simulink model "ev_control"  (R2024b)
settings: Solver=ode23t  StartTime=0  StopTime=3000  FixedStep=0.1  RelTol=1e-3
undefined symbols (not defined in the file or in its folder): DiscIntNeverNeededParam, Ion, Lithium
libraries: fl_lib x7, nesl_utility x7, sdl_lib x6, autolibshared x5, ee_lib x3, spsBatteryLib x1, spsControlledCurrentSourceLib x1, rllib x1, spspowerguiLib x1
settings Model: Creator=aaksh  LastModifiedBy=CSLAB

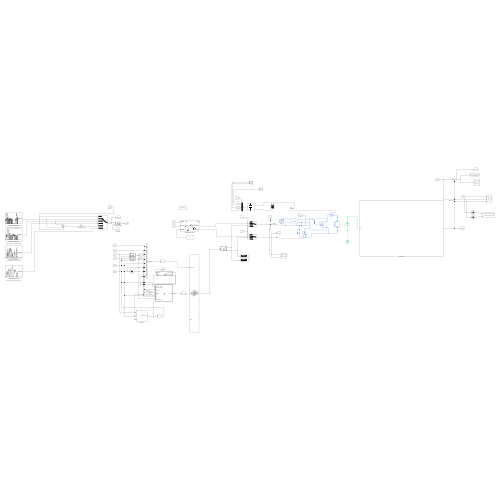
[thumbnail: Simulink's stored preview of the top-level diagram]
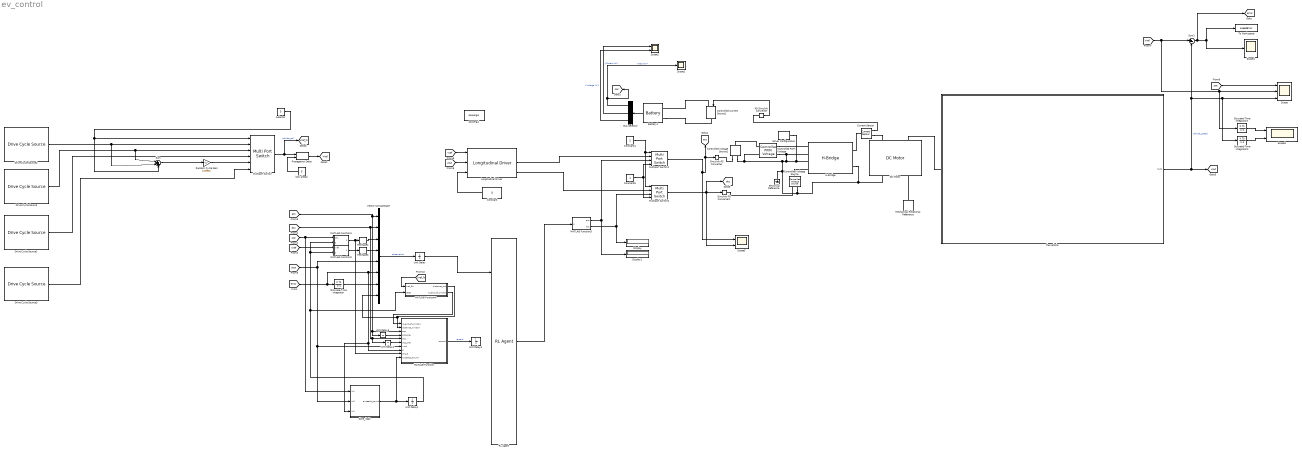
== system ev_control ==
  Battery1 : spsBatteryLib/Battery  BatType=Lithium-Ion  NomV=360  NomQ=77  SOC=76.3292  Batt_Tr=30  PresetModel=on  MaxQ=77  MinV=270  FullV=419.0354  Dis_rate=33.4783  R=0.046753  Normal_OP=69.6348  expZone="[388.9389      3.783043]"
      settings: LibrarySourceBlock=electricdrivelib/Extra Sources/Battery
  Bus Selector : BusSelector  OutputSignals=SOC (%),Current (A),Voltage (V)
  Constant : Constant  Value=0
  Constant4 : Constant  Value=2
  Constant5 : Constant
  Controlled Current Source1 : spsControlledCurrentSourceLib/Controlled Current Source  Initialize=on  Source_Type=AC  Amplitude=0  Phase=0  Frequency=0  Measurements=None
  Controlled PWM Voltage : ee_lib/Integrated Circuits/Controlled PWM Voltage  F=7 kHz  TD=0 s  pulse_width_offset=0 s  pulse_min=0 s  pwm_or_av=ee.enum.pwm_or_av.averaged  event_type=ee.enum.ic.event.asynchronous  sample_time=1e-6 s  Vmin=0 V  Vmax=1 V  Vm=1 V  u_min=0  u_max=1
  Controlled Voltage Source : fl_lib/Electrical/Electrical Sources/Controlled Voltage Source
  Controlled Voltage Source1 : fl_lib/Electrical/Electrical Sources/Controlled Voltage Source
  Current Sensor : fl_lib/Electrical/Electrical Sensors/Current Sensor
  DC Motor : ee_lib/Electromechanical/Brushed Motors/DC Motor  field_option=ee.enum.field_option.pm  Rf=100 Ohm  Lf=1 H  Laf=0.15 H  If0=0 A  parameterization=ee.enum.dcparam_option.load_speed  Ra=3.9 Ohm  La=100e-6 H  emf_or_torque=ee.enum.emf_or_torque.kv  Kv=0.072e-3 V/rpm  Ki=6.876e-4 N*m/A  T_stall=0.24e-3 N*m  w_max=8000 rpm  w_rated=6000 rpm  P_rated=89 kW  V_rated=360 V  lam_param=ee.enum.lam_param.damping  i_noload=0 A  V_i_noload=1.5 V  J=0.03 kg*m^2  lam=0.02 N*m*s/rad  speed0=0 rpm  t_fault_armature=1 s  t_fault_field=1 s  fault_action=simscape.enum.assert.action.none  alpha=3.93e-3 1/K  Tmeas=25 degC  thermal_mass=100 J/K  initial_temperature=25 degC
  Discrete-Time Integrator : DiscreteIntegrator  SampleTime=-1  ICPrevOutput=DiscIntNeverNeededParam  ICPrevScaledInput=DiscIntNeverNeededParam
  Discrete-Time Integrator1 : DiscreteIntegrator  SampleTime=-1  ICPrevOutput=DiscIntNeverNeededParam  ICPrevScaledInput=DiscIntNeverNeededParam
  Discrete-Time Integrator2 : DiscreteIntegrator  SampleTime=-1  ICPrevOutput=DiscIntNeverNeededParam  ICPrevScaledInput=DiscIntNeverNeededParam
  Display : Display
  Display1 : Display
  Drive Cycle Source : autolibshared/Drive Cycle Source  cycleVar=FTP72  fileVar=cycleFTP75.mat  tfinal="1372  seconds, Cyclic"  cycleRepeat=on  outAccPort=off  outGearPort=off  gearList=No gear data  t_wot1=5  xdot_woto=0  xdot_wot1=30  t_wot2=20  xdot_wot2=0  t_wotend=30  srcUnit=m/s  outUnit=m/s  srcAccUnit=m/s/s  outAccUnit=m/s^2  dt=0.1  aMode=1  faultOption=off  velBnd=2  velBndUnit=mph  inUnit=m/s  timeBnd=1  failOption=off  stopSim=off  maxFaultCnt=10  maxFaultTime=2  maxTotFaultTime=15  traceOption=off  dtTrace=1  traceWindow=10  lastDCname=FTP72  lastOutUnit=mph  lastDT=0  lastTB=1  lastSB=2  forceCalcBound=off
  Drive Cycle Source1 : autolibshared/Drive Cycle Source  cycleVar=NYCC  fileVar=cycleFTP75.mat  tfinal="598  seconds, Cyclic"  cycleRepeat=on  outAccPort=off  outGearPort=off  gearList=No gear data  t_wot1=5  xdot_woto=0  xdot_wot1=30  t_wot2=20  xdot_wot2=0  t_wotend=30  srcUnit=m/s  outUnit=m/s  srcAccUnit=m/s/s  outAccUnit=m/s^2  dt=0.1  aMode=1  faultOption=off  velBnd=2  velBndUnit=mph  inUnit=m/s  timeBnd=1  failOption=off  stopSim=off  maxFaultCnt=10  maxFaultTime=2  maxTotFaultTime=15  traceOption=off  dtTrace=1  traceWindow=10  lastDCname=NYCC  lastOutUnit=mph  lastDT=0  lastTB=1  lastSB=2  forceCalcBound=off
  Drive Cycle Source2 : autolibshared/Drive Cycle Source  cycleVar=FTP75  fileVar=cycleFTP75.mat  tfinal="2474  seconds, Cyclic"  cycleRepeat=on  outAccPort=off  outGearPort=off  gearList=No gear data  t_wot1=5  xdot_woto=0  xdot_wot1=30  t_wot2=20  xdot_wot2=0  t_wotend=30  srcUnit=m/s  outUnit=m/s  srcAccUnit=m/s/s  outAccUnit=m/s^2  dt=0.1  aMode=1  faultOption=off  velBnd=2  velBndUnit=mph  inUnit=m/s  timeBnd=1  failOption=off  stopSim=off  maxFaultCnt=10  maxFaultTime=2  maxTotFaultTime=15  traceOption=off  dtTrace=1  traceWindow=10  lastDCname=FTP75  lastOutUnit=mph  lastDT=0  lastTB=1  lastSB=2  forceCalcBound=off
  Drive Cycle Source3 : autolibshared/Drive Cycle Source  cycleVar=SC03  fileVar=cycleFTP75.mat  tfinal="600  seconds, Cyclic"  cycleRepeat=on  outAccPort=off  outGearPort=off  gearList=No gear data  t_wot1=5  xdot_woto=0  xdot_wot1=30  t_wot2=20  xdot_wot2=0  t_wotend=30  srcUnit=m/s  outUnit=m/s  srcAccUnit=m/s/s  outAccUnit=m/s^2  dt=0.1  aMode=1  faultOption=off  velBnd=2  velBndUnit=mph  inUnit=m/s  timeBnd=1  failOption=off  stopSim=off  maxFaultCnt=10  maxFaultTime=2  maxTotFaultTime=15  traceOption=off  dtTrace=1  traceWindow=10  lastDCname=SC03  lastOutUnit=mph  lastDT=0  lastTB=1  lastSB=2  forceCalcBound=off
  Electrical Reference : fl_lib/Electrical/Electrical Elements/Electrical Reference
  H-Bridge : ee_lib/Semiconductors & Converters/Converters/H-Bridge  supply_ports=ee.enum.supply_ports.hidesupply  pwm_or_av=ee.enum.pwm_or_av.averaged  regenerative_braking_mode=ee.enum.converters.regenerative_braking_mode.always_enabled  discontinuous=ee.enum.current_profile.continuous  freewheeling_mode=ee.enum.converters.freewheeling_mode.one_switch_one_diode  Rload=10 Ohm  Lload=1e-5 H  F=10 kHz  Venable=0.001 V  Vmax=1 V  Vreverse=0.001 V  Vbrake=0.001 V  Vm=360 V  Ron=0.1 Ohm  Don=0.05 Ohm  Goff=1e-6 S  Tmeas=298.15 K  Ron2=0.1 Ohm  Don2=0.05 Ohm  Tmeas2=398.15 K  thermal_mass=100 J/K  initial_temperature=298.15 K
  Longitudinal Driver : autolibshared/Longitudinal Driver  extAccelOvr=off  extDecelOvr=off  extAccelHld=off  extDecelHld=off  extAccelZero=off  extDecelZero=off  cntrlType=PI  shftType=None  velUnits=m/s  gearOut=off  Kp=60  Ki=5  Kff=.05  Kg=.01  VehVelVec=[0 100]  KffVec=[.1 .1]  KpVec=[10 10]  KiVec=[5 5]  KgVec=[0 0]  m=1500  Kpt=3000  tau=.1  L=2  aR=200  bR=2.5  cR=.5  g=9.81  vnom=30  Kaw=.1  tauerr=.03  tauPt=2  GearInit=0  tShift=.1  pdlVec=[0.1 0.4 0.5 0.9]  upShftTbl=[-1 12.9375 26.4375 39.9375 51.18749999999999 62.4375 72.84375 83.25;-1 16.3125 29.8125 43.3125 54.5624 65.8125 76.78125 87.75;-1 19.6875 33.1875 46.68749999999999 57.9375 69.1875 80.71875 92.25;-1 33 52.5 77.25 100.5 138.75 161.875 185]  dwnShftTbl=[1 9.5625 23.0625 36.5625 47.8125 59.0625 68.90625 78.75;1 12.9375 26.4375 39.9375 51.18749999999999 62.4375 72.84375 83.25;1 16.3125 29.8125 43.3125 54.562499 65.8125 76.78125 87.75;1 19.6875 33.1875 46.68749999999999 57.9375 69.1875 80.71875 92.25]  tClutch=.5  tRev=.5  tPark=120  aMode=1  UpGearVec="[0  1  2  3  4  5  6  7]"  DownGearVec="[1  2  3  4  5  6  7  8]"
  MATLAB Function : MATLAB Function  TreatAsAtomicUnit=on  SystemSampleTime=0.1
  MATLAB Function1 : MATLAB Function  TreatAsAtomicUnit=on  SystemSampleTime=0.1
  MATLAB Function2 : MATLAB Function  TreatAsAtomicUnit=on  SystemSampleTime=0.1
  MATLAB Function3 : MATLAB Function  TreatAsAtomicUnit=on
  MATLAB Function4 : MATLAB Function  TreatAsAtomicUnit=on  SystemSampleTime=0.1
  Mechanical Rotational Reference : fl_lib/Mechanical/Rotational Elements/Mechanical Rotational Reference
  Multiport Switch : MultiPortSwitch  Inputs=5  SaturateOnIntegerOverflow=off  InputSameDT=off
  Multiport Switch1 : MultiPortSwitch  SaturateOnIntegerOverflow=off  InputSameDT=off
  Multiport Switch2 : MultiPortSwitch  SaturateOnIntegerOverflow=off  InputSameDT=off
  PS-Simulink Converter : nesl_utility/PS-Simulink Converter  PhysicalDomain=network_engine_domain  SubClassName=ps_output  LeftPortType=input  RightPortType=output  PseudoPeriodic=off  Frequencies=[]  VectorFormat=inherit  Unit=inherit  AffineConversion=off
  Propagation Delay : PropagationDelay
  RL Agent : rllib/RL Agent  Agent=agent  ExternalActionAsInput=off  ProvideLastAction=off  ProvideCumRwd=off  TreatAsDirectFeedthrough=on  UseStrictObservationDataTypes=off
  Random Cycle Gain : Gain  Gain=0.29961
  Reshape2 : Reshape
  Reshape3 : Reshape
  Scope : Scope  NumInputPorts=3
  Scope1 : Scope
  Scope2 : Scope  NumInputPorts=2
  Scope3 : Scope  NumInputPorts=2
  Scope4 : Scope
  Scope5 : Scope  NumInputPorts=2
  Simulink-PS Converter : nesl_utility/Simulink-PS Converter  PhysicalDomain=network_engine_domain  SubClassName=ps_input  LeftPortType=input  RightPortType=output  PseudoPeriodic=off  Frequencies=[]  NoiseDistribution=none  NoiseParameters=[]  Unit=1  AffineConversion=off  FilteringAndDerivatives=filter  SimscapeFilterOrder=1  InputFilterTimeConstant=0.1  UdotUserProvided=0
  Simulink-PS Converter1 : nesl_utility/Simulink-PS Converter  PhysicalDomain=network_engine_domain  SubClassName=ps_input  LeftPortType=input  RightPortType=output  PseudoPeriodic=off  Frequencies=[]  NoiseDistribution=none  NoiseParameters=[]  Unit=1  AffineConversion=off  FilteringAndDerivatives=filter  SimscapeFilterOrder=1  InputFilterTimeConstant=0.1  UdotUserProvided=0
  Solver Configuration : nesl_utility/Solver Configuration  PhysicalDomain=network_engine_domain  SubClassName=solver  LeftPortType=input  RightPortType=generic  Tones=[]  Harmonics=[]  SimulateNoise=off  Profile=off  UseLocalSampling=off  EnableSwitchedLinearOptims=on  FrequencyDomain=off  UseCCode=off  RelTol=0.001  AbsTol=0.001  MinStep=1e-09  ToWorkspace=off  RevertToSquareIcSolve=off  NumHomotopyIterations=100  PhasorMode=off  PhasorModeNumHarmonics=1  ConsistencySolver=NEWTON_XTOL_AFTER_FTOL  IndexReductionMethod=DerivativeReplacement  DoDC=off  ResidualTolerance=1e-09  ConsistencyTolSource=GLOBAL  ConsistencyAbsTol=0.001  ConsistencyRelTol=0.001  ConsistencyTolFactor=0.001  UseLocalSolver=off  LocalSolverChoice=NE_BACKWARD_EULER_ADVANCER  ResolveIndetEquations=on  FunctionEvalNumThread=1  LocalSolverSampleTime=0.001  DoFixedCost=off  MaxNonlinIter=3  MaxModeIter=2  ComputeImpulses=off  ImpulseIterations=2  LinearAlgebra=auto  LinearAlgebraNumThread=0  EquationFormulation=NE_TIME_EF  DelaysMemoryBudget=2048  AutomaticFiltering=on  FilteringTimeConstant=0.01  PartitionStorageMethod=AS_NEEDED  PartitionMemoryBudget=1024  PartitionMethod=ROBUST  MultibodyUseLocalSolver=off  MultibodyLocalSolverChoice=ODE1  MultibodyLocalSolverSampleTime=0.001
  Sum : Sum  Inputs=|+++
  Sum1 : Sum  Inputs=|+-
  To Workspace : ToWorkspace  VariableName=speedError  SampleTime=-1
  Unit Delay{,1..4} (5 alike) : UnitDelay  SampleTime=-1  HasFrameUpgradeWarning=on
  Vector Concatenate : Concatenate  NumInputs=8
  done_logic : Subsystem
  look ahead : Constant  Value=5
  powergui : spspowerguiLib/powergui  Priority=1  SimulationMode=Continuous  SampleTime=50e-6  frequency=60  Iterations=50  frequencyindice=0  Pbase=100e6  ErrMax=1e-4  UnitsV=kV  UnitsW=MW  buscounter=0  FunctionMessages=off  echomessages=off  EnableUseOfTLC=off  CurrentSourceSwitches=off  DisableSnubberDevices=off  DisableRonSwitches=off  DisableVfSwitches=off  DisplayEquations=off  AutomaticDiscreteSolvers=off  SolverType=Tustin/Backward Euler (TBE)  Interpol=off  ExternalGateDelay=off  methode=off  Ts=100  x0status=blocks  SPID=on  SwTol=0  HookPort=off  NonlinearTolerance=1e-4  nMaxIteration=100  ContinueOnMaxIteration=off  RestoreLinks=warning  ResistiveCurrentMeasurement=off  Frange=[0:2:500]  Ylog=off  Xlog=on  ShowGrid=off  save=off  variable=ZData  structure=0  ZoomFFT=off  StartTime=0.0  cycles=1  DisplayStyle=1  fundamental=60  FreqAxis=off  MaxFrequency=1000  frequencyindicesteady=1  RmsSteady=1  display=off
  selector : Constant  Value=5
  the vehicle : Subsystem
  tag scope: Vref=global, Vref_lh=global, acc=global, dcc=global, error=global, soc=global, vout=global
  wires:
  the vehicle/1(Out1) -> Sum1/2, Discrete-Time Integrator2/1, Scope/3, [vout]  "vehicle_speed"
  Constant/1 -> Longitudinal Driver/3
  Drive Cycle Source/1 -> Multiport Switch/3, Sum/1
  Multiport Switch/1 -> [Vref_lh], Propagation Delay/1  "vehicle_ref"
  selector/1 -> Sum/3, Multiport Switch/1
  PS-Simulink Converter/1 -> Controlled Current Source1/1
  Battery1/1 -> Bus Selector/1
  Bus Selector/1 -> Scope1/1, [soc]  "<SOC (%)>"
  Bus Selector/2 -> Scope2/1  "<Current (A)>"
  Bus Selector/3 -> Scope2/2  "<Voltage (V)>"
  Sum1/1 -> [error], To Workspace/1, Scope4/1
  Longitudinal Driver/3 -> Multiport Switch2/2
  Longitudinal Driver/2 -> Multiport Switch1/2
  Constant4/1 -> Multiport Switch2/1, Multiport Switch1/1
  Constant5/1 -> Multiport Switch2/4, Multiport Switch1/4
  [error] -> done_logic/3(In2), MATLAB Function/8(e), Vector Concatenate/6, Discrete-Time Integrator/1
  [soc] -> done_logic/1(In1), MATLAB Function1/1(soc)
  [vout] -> done_logic/2(In3), MATLAB Function/7(vout), Vector Concatenate/5
  Discrete-Time Integrator/1 -> Vector Concatenate/7
  MATLAB Function1/1(soc_5) -> MATLAB Function/9(soc_5), Reshape2/1
  MATLAB Function2/1(vref_5) -> Reshape3/1
  [Vref] -> MATLAB Function2/1(vref)
  done_logic/1(exceeds_bound) -> Unit Delay1/1, MATLAB Function/10(exceeds_bound)
  Drive Cycle Source1/1 -> Multiport Switch/4
  Drive Cycle Source2/1 -> Sum/2, Multiport Switch/2
  Reshape2/1 -> Vector Concatenate/3
  Reshape3/1 -> Vector Concatenate/4
  Vector Concatenate/1 -> Unit Delay/1  "observation"
  Unit Delay/1 -> RL Agent/1
  MATLAB Function3/1(acc) -> Multiport Switch1/3, Display1/1
  MATLAB Function3/2(dcc) -> Multiport Switch2/3, Display/1
  RL Agent/1 -> MATLAB Function3/1(a)
  Unit Delay1/1 -> MATLAB Function4/2(reset), MATLAB Function1/2(reset), MATLAB Function2/2(reset)
  MATLAB Function/1(reward) -> Unit Delay2/1  "reward"
  Multiport Switch1/1 -> Scope5/1, [acc], Simulink-PS Converter/1
  Multiport Switch2/1 -> [dcc], Scope5/2, Simulink-PS Converter1/1
  Drive Cycle Source3/1 -> Multiport Switch/6
  [dcc] -> Vector Concatenate/2, MATLAB Function/5(dcc), Unit Delay4/1
  [acc] -> Vector Concatenate/1, Unit Delay3/1, MATLAB Function/3(acc)
  Unit Delay3/1 -> MATLAB Function/4(acc_prev)
  Unit Delay4/1 -> MATLAB Function/6(dcc_prev)
  Sum/1 -> Random Cycle Gain/1
  Random Cycle Gain/1 -> Multiport Switch/5
  [Vref] -> Longitudinal Driver/1
  [Vref] -> Discrete-Time Integrator1/1, Scope/2, Sum1/1
  [vout] -> Longitudinal Driver/2
  Propagation Delay/1 -> [Vref]
  look ahead/1 -> Propagation Delay/2
  [soc] -> Scope/1
  [Vref_lh] -> MATLAB Function4/1(vref_50)
  MATLAB Function4/1(distance_out) -> MATLAB Function/2(distance_window), Vector Concatenate/8
  MATLAB Function4/2(is_end_of_window) -> MATLAB Function/1(is_end_of_window)
  Discrete-Time Integrator1/1 -> Scope3/1
  Discrete-Time Integrator2/1 -> Scope3/2
  connections:
  DC Motor/LConn2 -- the vehicle/LConn1
  Mechanical Rotational Reference/LConn1 -- DC Motor/RConn2
  H-Bridge/RConn1 -- Current Sensor/LConn1
  Controlled PWM Voltage/RConn2 -- Solver Configuration/RConn1 -- H-Bridge/LConn3 -- Controlled Voltage Source1/RConn2 -- Controlled PWM Voltage/LConn2 -- Electrical Reference/LConn1 -- Controlled Voltage Source/RConn2 -- H-Bridge/RConn2 -- DC Motor/RConn1 -- H-Bridge/LConn2
  Controlled PWM Voltage/RConn1 -- H-Bridge/LConn1
  Controlled PWM Voltage/LConn1 -- Controlled Voltage Source1/LConn1
  Controlled Voltage Source/LConn1 -- H-Bridge/LConn4
  Controlled Voltage Source1/RConn1 -- Simulink-PS Converter/RConn1
  Simulink-PS Converter1/RConn1 -- Controlled Voltage Source/RConn1
  Current Sensor/RConn2 -- DC Motor/LConn1
  Current Sensor/RConn1 -- PS-Simulink Converter/LConn1
  Battery1/LConn2 -- Controlled Current Source1/RConn1
  Controlled Current Source1/LConn1 -- Battery1/LConn1

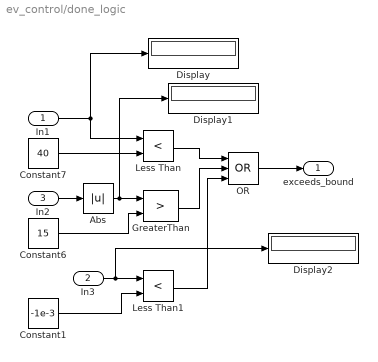
== system ev_control/done_logic ==
  In1 : Inport
  In3 : Inport  Port=2
  In2 : Inport  Port=3
  Abs : Abs  SaturateOnIntegerOverflow=off
  Constant1 : Constant  Value=-1e-3
  Constant6 : Constant  Value=15
  Constant7 : Constant  Value=40
  Display : Display
  Display1 : Display
  Display2 : Display
  GreaterThan : RelationalOperator  Operator=>  OutDataTypeStr=boolean  RndMeth=Simplest  InputSameDT=off
  Less Than : RelationalOperator  Operator=<  OutDataTypeStr=boolean  RndMeth=Simplest  InputSameDT=off
  Less Than1 : RelationalOperator  Operator=<  OutDataTypeStr=boolean  RndMeth=Simplest  InputSameDT=off
  OR : Logic  Operator=OR  Inputs=3  IconShape=distinctive  AllPortsSameDT=off  OutDataTypeStr=boolean
  exceeds_bound : Outport
  wires:
  GreaterThan/1 -> OR/2
  Constant6/1 -> GreaterThan/2
  Less Than/1 -> OR/1
  Abs/1 -> GreaterThan/1, Display1/1
  OR/1 -> exceeds_bound/1
  In1/1 -> Less Than/1, Display/1
  Constant7/1 -> Less Than/2
  In2/1 -> Abs/1
  In3/1 -> Display2/1, Less Than1/1
  Constant1/1 -> Less Than1/2
  Less Than1/1 -> OR/3

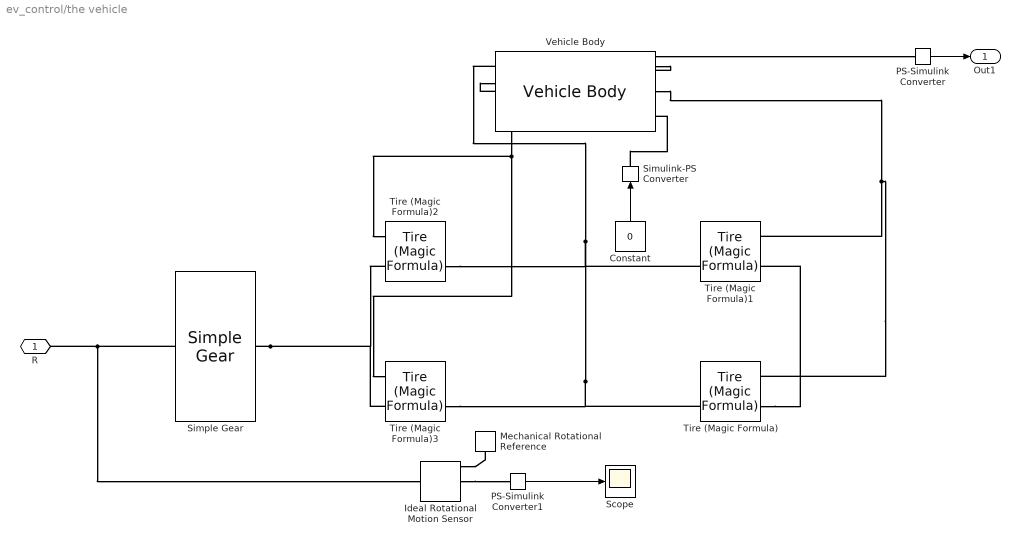
== system ev_control/the vehicle ==
  Constant : Constant  Value=0
  Ideal Rotational Motion Sensor : fl_lib/Mechanical/Mechanical Sensors/Ideal Rotational Motion Sensor  reference=foundation.enum.MeasurementReference.difference  acceleration_port=false  velocity_port=true  position_port=true  wrap_angle=false  offset=0 rev
  Mechanical Rotational Reference : fl_lib/Mechanical/Rotational Elements/Mechanical Rotational Reference
  PS-Simulink Converter : nesl_utility/PS-Simulink Converter  PhysicalDomain=network_engine_domain  SubClassName=ps_output  LeftPortType=input  RightPortType=output  PseudoPeriodic=off  Frequencies=[]  VectorFormat=inherit  Unit=inherit  AffineConversion=off
  PS-Simulink Converter1 : nesl_utility/PS-Simulink Converter  PhysicalDomain=network_engine_domain  SubClassName=ps_output  LeftPortType=input  RightPortType=output  PseudoPeriodic=off  Frequencies=[]  VectorFormat=inherit  Unit=inherit  AffineConversion=off
  Scope : Scope
  Simple Gear : sdl_lib/Gears/Simple Gear  ratio=7  rotation_direction=sdl.enum.shaftOutputDirection.same  friction_model=sdl.enum.gear_efficiencies_load.off  T_noload=0.1 N*m  T_nom=5 N*m  efficiency_nom=0.8  efficiency=0.8  temperature_TLU=[280, 300, 320] K  load_TLU=[1, 5, 10] N*m  efficiency_TLU=[.95, .9, .85]  efficiency_TLU2=[.85, .8, .75; .95, .9, .85; .85, .8, .7]  w_thr=0.01 rad/s  pwr_thr=0.001 W  enable_backlash=false  hardstop_model=simscape.enum.hardstop.smooth  backlash_distance=1e-3 mm  r_base=0.1 m  transition=1e-4 mm  backlash_stiffness=1e6 N/m  backlash_damping=1e3 N*s/m  coeff_rest=0.7  v_tol=0.001 m/s  f_tol=0.001 N  mu_visc=[0, 0] N*m*s/rad  thermal_mass=50 J/K  temperature_specify=off  temperature_priority=High  temperature=300 K  temperature_nominal_specify=off  temperature_nominal_value=1  temperature_nominal_unit=K  x_backlash_specify=off  x_backlash_priority=None  x_backlash=0 mm  x_backlash_nominal_specify=off  x_backlash_nominal_value=1  x_backlash_nominal_unit=mm  f_hardstop_specify=off  f_hardstop_priority=None  f_hardstop=0 N  f_hardstop_nominal_specify=off  f_hardstop_nominal_value=1  f_hardstop_nominal_unit=N  v_backlash_specify=off  v_backlash_priority=None  v_backlash=0 m/s  v_backlash_nominal_specify=off  v_backlash_nominal_value=1  v_backlash_nominal_unit=m/s
  Simulink-PS Converter : nesl_utility/Simulink-PS Converter  PhysicalDomain=network_engine_domain  SubClassName=ps_input  LeftPortType=input  RightPortType=output  PseudoPeriodic=off  Frequencies=[]  NoiseDistribution=none  NoiseParameters=[]  Unit=1  AffineConversion=off  FilteringAndDerivatives=provide  SimscapeFilterOrder=1  InputFilterTimeConstant=0.001  UdotUserProvided=0
  Tire (Magic Formula){,1..3} (4 alike) : sdl_lib/Tires & Vehicles/Tire (Magic Formula)  parameterization=sdl.enum.magic_tire_model.peak  F_z1=3000 N  F_x1=3500 N  kappa1=10  B_m=10  C_m=1.9  D_m=1  E_m=0.97  fz0=4000 N  p_Cx=1.685  p_Dx=[1.21, -.037]  p_Ex=[.344, .095, -.02, 0]  p_Kx=[21.51, -.163, .245]  p_Hx=[-.002, .002]  p_Vx=[0, 0]  rolling_radius_model=sdl.enum.RollingRadiusParameterization.Constant  r_e=0.3 m  r_0=0.3 m  breff=8.39  dreff=0.26  freff=0.074  q_re0=0.99  q_v1=0.008  longvl=17 m/s  cz=5e5 N/m  model_resistance=false  resistance_model=sdl.enum.rollingResistanceParameterization.constant  coeff=0.015  p_tire=250e3 Pa  alpha=-0.003  beta=0.97  coeff_a=84e-4  coeff_b=6.2e-4 s/m  coeff_c=1.6e-4 s^2/m^2  p_tire0=240e3 Pa  fz0_resistance=4000 N  vH0=16 m/s  q_Sy=[.0082, 0, .0014, .001, 0, 0, 1.08, -.5]  v_thr=0.001 m/s  enable_scaling_coefficients=false  lfzO=1  lcx=1  lmux=1  lex=1  lkx=1  lhx=1  lvx=1  lmy=1  model_compliance=sdl.enum.compliance.off  stiffness=1e6 N/m  damping=1000 N*s/m  model_inertia=sdl.enum.model_inertia.off  inertia=1 kg*m^2  initial_velocity=0 rad/s  vxlow=1 m/s  v_tr_thr=0.1 m/s  kpumin=-1.5  kpumax=1.5
  Vehicle Body : sdl_lib/Tires & Vehicles/Vehicle Body  mass=1200 kg  n_w=2  x_f=1.4 m  x_r=1.6 m  y_c=0.5 m  mass_var=false  g=9.81 m/s^2  liftoff_warning=false  area=3 m^2  Cd_var=false  Cd=0.4  rho=1.18 kg/m^3  model_pitch=false  inertia=4000 kg*m^2  suspension_model=sdl.enum.linearTLU.linear  k_f=1e4 N/m  b_f=1e4 N*s/m  k_r=1e4 N/m  b_r=1e4 N*s/m  k_f_TLU=[-2000, -1000, 0, 1000, 2000] N  x_f_TLU=[-.4, -.2, 0, .2, .4] m  b_f_TLU=[-200, -100, 0, 100, 200] N  v_f_TLU=[-4, -2, 0, 2, 4] m/s  k_r_TLU=[-2000, -1000, 0, 1000, 2000] N  x_r_TLU=[-.4, -.2, 0, .2, .4] m  b_r_TLU=[-200, -100, 0, 100, 200] N  v_r_TLU=[-4, -2, 0, 2, 4] m/s  interp_method=simscape.enum.interpolation.linear  extrap_method=simscape.enum.extrapolation.linear  model_hardstop=false  upper_bound_f=.25 m  lower_bound_f=-.25 m  stop_k_f=1e6 N/m  stop_b_f=150 N*s/m  upper_bound_r=.25 m  lower_bound_r=-.25 m  stop_k_r=1e6 N/m  stop_b_r=150 N*s/m  initial_pitch=0 rad  initial_pitch_rate=0 rad/s  v_specify=off  v_priority=Low  v=0 m/s  v_nominal_specify=off  v_nominal_value=1  v_nominal_unit=m/s
      settings: InternalSimscapePortConfiguration="{\"Bottom\":[{\"id\":\"NR\",\"label\":\"NR\",\"type\":\"output\"},{\"id\":\"NF\",\"label\":\"NF\",\"type\":\"output\"},{\"id\":\"beta\",\"label\":\"beta\",\"type\":\"input\"}],\"Left\":[{\"id\":\"H\",\"label\":\"H\",\"type\":\"foundation.mechanical.translational.translational\"}],\"Right\":[],\"Top\":[{\"id\":\"V\",\"label\":\"V\",\"type\":\"output\"},{\"id\":\"wind\",\"label\":\"W\",\"type\":\"input\"}]}"
  R : PMIOPort  Side=Left
  Out1 : Outport
  wires:
  PS-Simulink Converter/1 -> Out1/1
  Constant/1 -> Simulink-PS Converter/1
  PS-Simulink Converter1/1 -> Scope/1
  connections:
  Tire (Magic Formula)/LConn2 -- Tire (Magic Formula)1/LConn2
  Vehicle Body/LConn1 -- Tire (Magic Formula)2/RConn2 -- Tire (Magic Formula)1/RConn2 -- Tire (Magic Formula)3/RConn2 -- Tire (Magic Formula)/RConn2
  Simple Gear/LConn1 -- Ideal Rotational Motion Sensor/LConn1 -- R/RConn1
  Simple Gear/RConn1 -- Tire (Magic Formula)2/LConn2 -- Tire (Magic Formula)3/LConn2
  Vehicle Body/LConn2 -- PS-Simulink Converter/LConn1
  Simulink-PS Converter/RConn1 -- Vehicle Body/RConn3
  Ideal Rotational Motion Sensor/RConn1 -- Mechanical Rotational Reference/LConn1
  Ideal Rotational Motion Sensor/RConn2 -- PS-Simulink Converter1/LConn1
  Vehicle Body/RConn2 -- Tire (Magic Formula)1/LConn1 -- Tire (Magic Formula)/LConn1
  Vehicle Body/RConn1 -- Tire (Magic Formula)3/LConn1 -- Tire (Magic Formula)2/LConn1

== matlab function ev_control/MATLAB Function1 ==
  data: soc input; soc_5 output size=[5 1]; reset input
% Change the function definition to accept two inputs
function soc_5 = fcn(soc, reset)

persistent data_soc;

% Update the condition to reset if the buffer is empty OR if reset is triggered
if isempty(data_soc) || reset == 1
    data_soc = zeros(5,1);
end

data_soc  = [soc; data_soc(1:4)];
soc_5 = data_soc;

end

== matlab function ev_control/MATLAB Function ==
  data: is_end_of_window input; distance_window input; acc input; acc_prev input; dcc input; dcc_prev input; vout input; e input; reward output; soc_5 input; exceeds_bound input
function reward = fcn(is_end_of_window, distance_window, acc, acc_prev, dcc, dcc_prev, vout, e, soc_5, exceeds_bound)
% REWARD FUNCTION FOR DISTANCE-WINDOW TRACKING (DUAL-COMMAND VERSION)
%
% INPUTS: (Matching the original block's wiring)
%   is_end_of_window: Flag (true if at the end of a 50-step window).
%   distance_window:  Target distance to cover in the 50-step window (m).
%   acc:              Current acceleration command [0, 1].
%   acc_prev:         Previous acceleration command [0, 1].
%   dcc:              Current deceleration command [0, 1].
%   dcc_prev:         Previous deceleration command [0, 1].
%   vout:             Current vehicle speed (m/s).
%   e:                Current speed error (Vref - Vout).
%   soc_5:            Vector of the 5 most recent SOC values.
%   exceeds_bound:    Flag (true if episode terminates for a fault).

    % --- 1. Define Constants & Weights ---
    Ts = 0.1;           % Model sample time
    MAX_STEPS = 30000;  % Total steps for normalization (as in original code)
    
    w_distance = 25.0;   % MAJOR penalty for distance tracking error
    w_velocity = 0.2;   % MINOR penalty for instantaneous velocity error
    w_soc      = 0.5;   % Penalty for deviating from the SOC comfort zone
    w_jerk     = 1.5;   % Penalty for jerky actions to encourage smoothness

    % --- 2. Accumulate Actual Distance Traveled ---
    persistent accumulated_distance;
    if isempty(accumulated_distance)
        accumulated_distance = 0;
    end
    accumulated_distance = accumulated_distance + (vout * Ts);

    % --- 3. Calculate Penalties ---

    % MAJOR PENALTY: Distance Tracking (applied only at the end of the window)
    distance_penalty = 0;
    if is_end_of_window
        distance_error = distance_window - accumulated_distance;
        distance_penalty = -w_distance * (distance_error^2);
        accumulated_distance = 0; % Reset for the next window
    end

    % MINOR PENALTY: Instantaneous Speed Tracking
    velocity_penalty = -w_velocity * (e^2);

    % SOC Penalty (maintains SOC between 60% and 90%)
    current_soc = soc_5(1); % CORRECTED: Use the first element, not the sum
    soc_upper_limit = 90.0;
    soc_lower_limit = 60.0;
    soc_penalty = 0;
    if current_soc > soc_upper_limit
        soc_penalty = -w_soc * (current_soc - soc_upper_limit)^2;
    elseif current_soc < soc_lower_limit
        soc_penalty = -w_soc * (soc_lower_limit - current_soc)^2;
    end
    
    % Jerk Penalty (using separate acc/dcc signals as requested)
    acc_jerk = acc - acc_prev;
    dcc_jerk = dcc - dcc_prev;
    jerk_penalty = -w_jerk * (acc_jerk^2 + dcc_jerk^2);

    % Boundary Penalty (for catastrophic failure)
    boundary_penalty = 0;
    if exceeds_bound > 0
        boundary_penalty = -1000;
    end

    % --- 4. Normalize and Calculate Total Reward ---
    % Normalizing the step-wise penalties as in your original function
    step_wise_penalties = distance_penalty + velocity_penalty + soc_penalty + jerk_penalty;
    normalized_reward = step_wise_penalties / MAX_STEPS;

    % Final reward includes the large boundary penalty and a small "living bonus"
    reward = normalized_reward + boundary_penalty + 0.1 + 0.001*vout;
end

== matlab function ev_control/MATLAB Function2 ==
  data: vref input; vref_5 output; reset input
% Change the function definition to accept two inputs
function vref_5 = fcn(vref, reset)

persistent data_vref;

% Update the condition to reset if the buffer is empty OR if reset is triggered
if isempty(data_vref) || reset == 1
    data_vref = zeros(5,1);
end

data_vref  = [vref; data_vref(1:4)];
vref_5 = data_vref;

end

== matlab function ev_control/MATLAB Function3 ==
  data: a input; acc output; dcc output
function [acc , dcc] = fcn(a)
act = a(1);
if act >= 0
    acc = abs(act);
    dcc = 0;
else
    acc = 0;
    dcc = abs(act);
end

== matlab function ev_control/MATLAB Function4 ==
  data: vref_50 input; distance_out output; reset input; is_end_of_window output
% Change the function definition to accept two inputs
function [distance_out, is_end_of_window]= fcn(vref_50, reset)

persistent data_window;
persistent counter;

ts = 0.1;

is_end_of_window = 0;
distance_out = 0;
% Update the condition to reset if the buffer is empty OR if reset is triggered
if isempty(data_window) || reset == 1
    data_window = zeros(50,1);
end

if isempty(counter)
        counter = 0;
end

counter = counter + 1;
data_window  = [vref_50; data_window(1:49)];

if counter >= 50
    distance_out = sum(data_window)*ts;
    is_end_of_window = 1;
    counter = 0;
end

end
